simulink model "bh_4dof_LAGR_manipulator_CONTROL_PID"  (R2016b)
settings: Solver=ode15s  StartTime=0.0  StopTime=60  FixedStep=0.001  RelTol=1e-5  EnableMultiTasking=on
values from neighbouring files (symbols this model uses):
  N = 3    [bh_4dof_sim_post_process.m]
undefined symbols (not defined in the file or in its folder): b1_damp, b2_damp, b3_damp, b4_damp, g, Hz, L1x, L1y, L1z, L2x, L2y, L2z, L3x, L3y, L3z, mass1, mass2, mass3, mass4, Rturn, theta1_0, theta1_dot_0, theta2_0, theta2_dot_0, theta3_0, theta3_dot_0, theta4_0, theta4_dot_0, X, Y, Z
libraries: sm_lib x25, nesl_utility x17, simulink x9, simulink_extras x2
(part 1 of 3)
settings Model: Creator=bhorton  LastModifiedBy=bhorton
settings SolverCC: ZeroCrossAlgorithm=Adaptive
settings OptimizationCC: LifeSpan=inf
settings DebuggingCC: SFUnexpectedBacktrackingDiag=warning  SFNoUnconditionalDefaultTransitionDiag=warning  SFExecutionAtInitializationDiag=none
settings GRTTargetCC: TargetLangStandard=C89/C90 (ANSI)
settings ConfigComp: CovMetricSettings=dw  CovHtmlReporting=on  CovSaveCumulativeToWorkspaceVar=on  CovSaveSingleToWorkspaceVar=on  CovExternalEMLEnable=off
settings SimscapeCC: SimscapeLogType=all  SimscapeLogDataHistory=10000

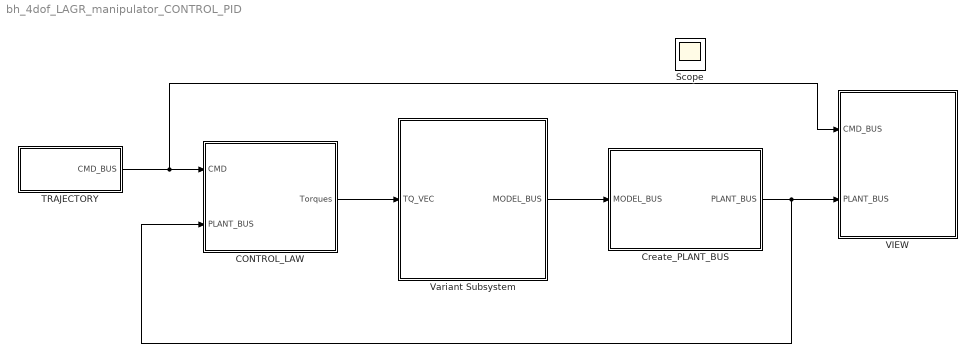
== system bh_4dof_LAGR_manipulator_CONTROL_PID ==
  CONTROL_LAW : Subsystem
  Create_PLANT_BUS : Subsystem
  TRAJECTORY : Subsystem
  VIEW : Subsystem
  Variant Subsystem : Subsystem  Variant=on  OverrideUsingVariant=Variant
  Scope : Scope
  wires:
  TRAJECTORY/1(CMD_BUS) -> VIEW/1(CMD_BUS), CONTROL_LAW/1(CMD)
  Create_PLANT_BUS/1(PLANT_BUS) -> VIEW/2(PLANT_BUS), CONTROL_LAW/2(PLANT_BUS)
  Variant Subsystem/1(MODEL_BUS) -> Create_PLANT_BUS/1(MODEL_BUS)
  CONTROL_LAW/1(Torques) -> Variant Subsystem/1(TQ_VEC)

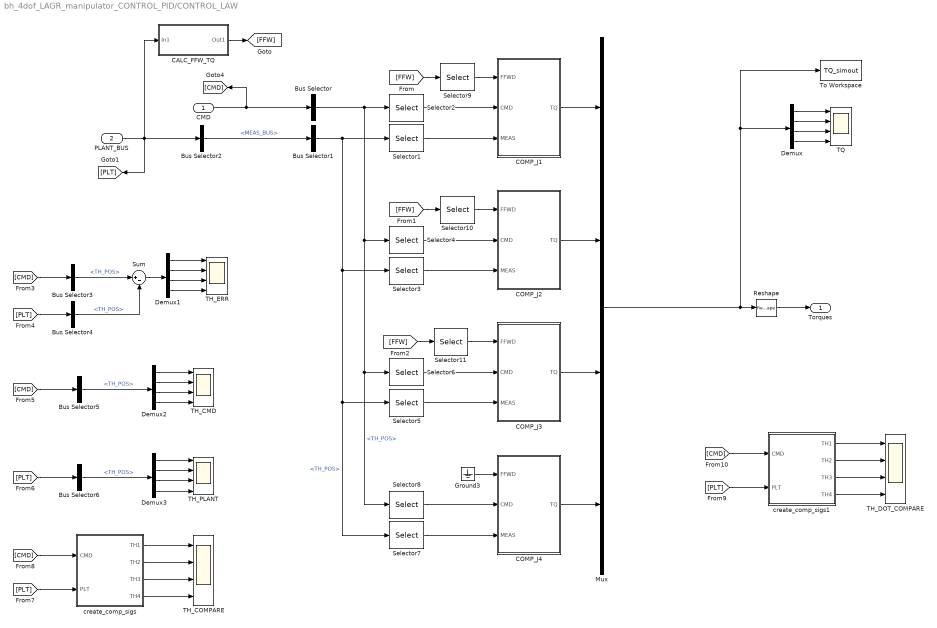
== system bh_4dof_LAGR_manipulator_CONTROL_PID/CONTROL_LAW ==
  CMD : Inport
  PLANT_BUS : Inport  Port=2
  Bus Selector{,1,3,5} (4 alike) : BusSelector  OutputSignals=TH_POS
  Bus Selector2 : BusSelector  OutputSignals=MEAS_BUS
  Bus Selector4 : BusSelector  OutputSignals=MEAS_BUS.TH_POS
  Bus Selector6 : BusSelector  OutputSignals=MEAS_BUS.TH_POS
  CALC_FFW_TQ : Subsystem
  COMP_J1 : Subsystem
  COMP_J2 : Subsystem
  COMP_J3 : Subsystem
  COMP_J4 : Subsystem
  Demux{,1..3} (4 alike) : Demux
  Ground3 : Ground
  Mux : Mux
  Reshape : Reshape  OutputDimensionality=Column vector (2-D)
  Selector1 : Selector  InputPortWidth=4  IndexOptions=Index vector (dialog)  Indices=1  OutputSizes=1
  Selector10 : Selector  InputPortWidth=3  IndexOptions=Index vector (dialog)  Indices=2  OutputSizes=1
  Selector11 : Selector  InputPortWidth=3  IndexOptions=Index vector (dialog)  Indices=3  OutputSizes=1
  Selector2 : Selector  InputPortWidth=4  IndexOptions=Index vector (dialog)  Indices=1  OutputSizes=1
  Selector3 : Selector  InputPortWidth=4  IndexOptions=Index vector (dialog)  Indices=2  OutputSizes=1
  Selector4 : Selector  InputPortWidth=4  IndexOptions=Index vector (dialog)  Indices=2  OutputSizes=1
  Selector5 : Selector  InputPortWidth=4  IndexOptions=Index vector (dialog)  Indices=3  OutputSizes=1
  Selector6 : Selector  InputPortWidth=4  IndexOptions=Index vector (dialog)  Indices=3  OutputSizes=1
  Selector7 : Selector  InputPortWidth=4  IndexOptions=Index vector (dialog)  Indices=4  OutputSizes=1
  Selector8 : Selector  InputPortWidth=4  IndexOptions=Index vector (dialog)  Indices=4  OutputSizes=1
  Selector9 : Selector  InputPortWidth=3  IndexOptions=Index vector (dialog)  Indices=1  OutputSizes=1
  Sum : Sum  Inputs=|+-
  TH_CMD : Scope  NumInputPorts=4
  TH_COMPARE : Scope  NumInputPorts=4
  TH_DOT_COMPARE : Scope  NumInputPorts=4
  TH_ERR : Scope  NumInputPorts=4
  TH_PLANT : Scope  NumInputPorts=4
  TQ : Scope  NumInputPorts=4
  To Workspace : ToWorkspace  VariableName=TQ_simout  SaveFormat=Structure With Time  SampleTime=-1
  create_comp_sigs : Subsystem
  create_comp_sigs1 : Subsystem
  Torques : Outport
  wires:
  Reshape/1 -> Torques/1
  Selector9/1 -> COMP_J1/1(FFWD)
  CMD/1 -> [CMD], Bus Selector/1
  Selector1/1 -> COMP_J1/3(MEAS)
  Selector2/1 -> COMP_J1/2(CMD)
  Bus Selector/1 -> Selector8/1, Selector6/1, Selector4/1, Selector2/1  "<TH_POS>"
  Bus Selector1/1 -> Selector5/1, Selector7/1, Selector3/1, Selector1/1  "<TH_POS>"
  Selector6/1 -> COMP_J3/2(CMD)
  Selector5/1 -> COMP_J3/3(MEAS)
  Selector3/1 -> COMP_J2/3(MEAS)
  Selector4/1 -> COMP_J2/2(CMD)
  Ground3/1 -> COMP_J4/1(FFWD)
  Selector8/1 -> COMP_J4/2(CMD)
  Selector7/1 -> COMP_J4/3(MEAS)
  COMP_J4/1(TQ) -> Mux/4
  COMP_J3/1(TQ) -> Mux/3
  COMP_J2/1(TQ) -> Mux/2
  COMP_J1/1(TQ) -> Mux/1
  Bus Selector2/1 -> Bus Selector1/1  "<MEAS_BUS>"
  Demux/1 -> TQ/1
  Demux/2 -> TQ/2
  Demux/4 -> TQ/4
  Demux/3 -> TQ/3
  CALC_FFW_TQ/1(Out1) -> [FFW]
  [FFW] -> Selector9/1
  [FFW] -> Selector10/1
  Selector10/1 -> COMP_J2/1(FFWD)
  [FFW] -> Selector11/1
  Selector11/1 -> COMP_J3/1(FFWD)
  Demux1/1 -> TH_ERR/1
  Demux1/2 -> TH_ERR/2
  Demux1/4 -> TH_ERR/4
  Demux1/3 -> TH_ERR/3
  PLANT_BUS/1 -> [PLT], CALC_FFW_TQ/1(In1), Bus Selector2/1
  [CMD] -> Bus Selector3/1
  [PLT] -> Bus Selector4/1
  Bus Selector3/1 -> Sum/1  "<TH_POS>"
  Bus Selector4/1 -> Sum/2  "<TH_POS>"
  Sum/1 -> Demux1/1
  Demux2/1 -> TH_CMD/1
  Demux2/2 -> TH_CMD/2
  Demux2/4 -> TH_CMD/4
  Demux2/3 -> TH_CMD/3
  [CMD] -> Bus Selector5/1
  Bus Selector5/1 -> Demux2/1  "<TH_POS>"
  Demux3/1 -> TH_PLANT/1
  Demux3/2 -> TH_PLANT/2
  Demux3/4 -> TH_PLANT/4
  Demux3/3 -> TH_PLANT/3
  [PLT] -> Bus Selector6/1
  Bus Selector6/1 -> Demux3/1  "<TH_POS>"
  [PLT] -> create_comp_sigs/2(PLT)
  [CMD] -> create_comp_sigs/1(CMD)
  create_comp_sigs/1(TH1) -> TH_COMPARE/1
  create_comp_sigs/2(TH2) -> TH_COMPARE/2
  create_comp_sigs/3(TH3) -> TH_COMPARE/3
  create_comp_sigs/4(TH4) -> TH_COMPARE/4
  [PLT] -> create_comp_sigs1/2(PLT)
  [CMD] -> create_comp_sigs1/1(CMD)
  create_comp_sigs1/1(TH1) -> TH_DOT_COMPARE/1
  create_comp_sigs1/2(TH2) -> TH_DOT_COMPARE/2
  create_comp_sigs1/3(TH3) -> TH_DOT_COMPARE/3
  create_comp_sigs1/4(TH4) -> TH_DOT_COMPARE/4
  Mux/1 -> To Workspace/1, Demux/1, Reshape/1

== system bh_4dof_LAGR_manipulator_CONTROL_PID/Create_PLANT_BUS ==
  MODEL_BUS : Inport
  CALC_BUS : Subsystem
  MEAS : Subsystem
  Subsystem : Subsystem
  Subsystem1 : Subsystem
  PLANT_BUS : Outport
  wires:
  MODEL_BUS/1 -> MEAS/1(MODEL_BUS), CALC_BUS/1(MODEL_BUS), Subsystem/1(MODEL)
  Subsystem/1(PLANT_B) -> PLANT_BUS/1
  CALC_BUS/1(CALC_POS) -> Subsystem1/1(POS), Subsystem/3(CALC_POS)
  MEAS/1(MEAS) -> Subsystem/2(MEAS)
  Subsystem1/1(GTQ) -> Subsystem/4(CALC_GRAV_TQ)

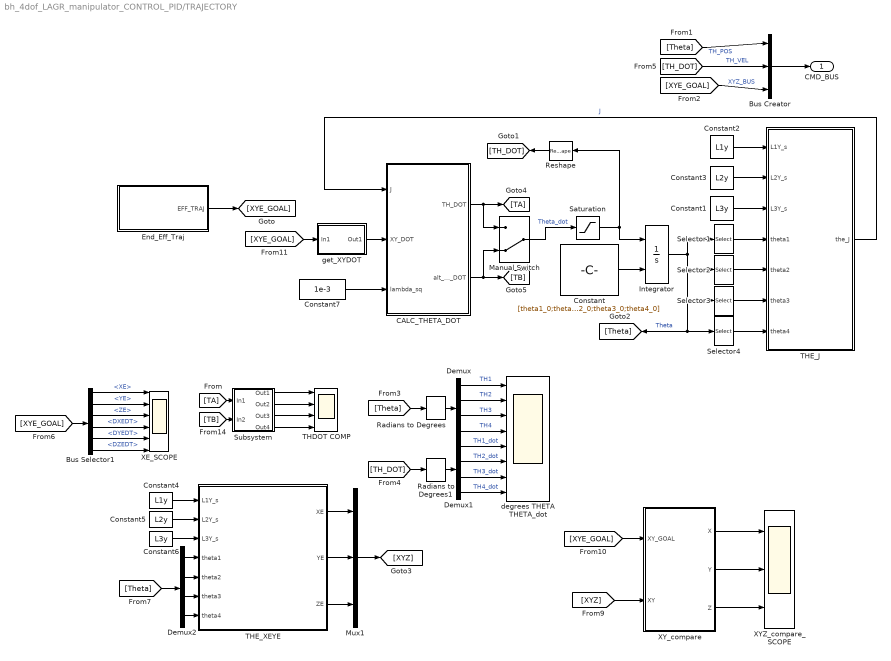
== system bh_4dof_LAGR_manipulator_CONTROL_PID/TRAJECTORY ==
  Bus Creator : BusCreator  Inputs=3
  Bus Selector1 : BusSelector  OutputSignals=XE,YE,ZE,DXEDT,DYEDT,DZEDT
  CALC_THETA_DOT : MATLAB Function  TreatAsAtomicUnit=on
  Constant : Constant  Value=[theta1_0;theta2_0;theta3_0;theta4_0]  VectorParams1D=off
  Constant1 : Constant  Value=L3y
  Constant2 : Constant  Value=L1y
  Constant3 : Constant  Value=L2y
  Constant4 : Constant  Value=L1y
  Constant5 : Constant  Value=L2y
  Constant6 : Constant  Value=L3y
  Constant7 : Constant  Value=1e-3
  Demux : Demux
  Demux1 : Demux
  Demux2 : Demux
  End_Eff_Traj : Subsystem
  Integrator : Integrator  InitialConditionSource=external
  Manual Switch : ManualSwitch  CurrentSetting=0
  Mux1 : Mux  Inputs=3
  Radians to Degrees : simulink_extras/Transformations/Radians to Degrees
  Radians to Degrees1 : simulink_extras/Transformations/Radians to Degrees
  Reshape : Reshape  OutputDimensionality=Column vector (2-D)
  Saturation : Saturate  UpperLimit=6  LowerLimit=-6
  Selector1 : Selector  InputPortWidth=4  IndexOptions=Index vector (dialog)  Indices=1  OutputSizes=1
  Selector2 : Selector  InputPortWidth=4  IndexOptions=Index vector (dialog)  Indices=2  OutputSizes=1
  Selector3 : Selector  InputPortWidth=4  IndexOptions=Index vector (dialog)  Indices=3  OutputSizes=1
  Selector4 : Selector  InputPortWidth=4  IndexOptions=Index vector (dialog)  Indices=4  OutputSizes=1
  Subsystem : Subsystem
  THDOT COMP : Scope  NumInputPorts=4
  THE_J : MATLAB Function  TreatAsAtomicUnit=on
  THE_XEYE : MATLAB Function  TreatAsAtomicUnit=on
  XE_SCOPE : Scope  NumInputPorts=6
  XYZ_compare_SCOPE : Scope  NumInputPorts=3
  XY_compare : Subsystem
  degrees THETA THETA_dot : Scope  NumInputPorts=8
  get_XYDOT : Subsystem
  CMD_BUS : Outport
  wires:
  Bus Selector1/1 -> XE_SCOPE/1  "<XE>"
  Bus Selector1/2 -> XE_SCOPE/2  "<YE>"
  Bus Selector1/3 -> XE_SCOPE/3  "<ZE>"
  Bus Selector1/4 -> XE_SCOPE/4  "<DXEDT>"
  Bus Selector1/5 -> XE_SCOPE/5  "<DYEDT>"
  Bus Selector1/6 -> XE_SCOPE/6  "<DZEDT>"
  [XYE_GOAL] -> Bus Selector1/1
  Constant/1 -> Integrator/2
  THE_J/1(the_J) -> CALC_THETA_DOT/1(J)  "J"
  get_XYDOT/1(Out1) -> CALC_THETA_DOT/2(XY_DOT)
  Manual Switch/1 -> Saturation/1  "Theta_dot"
  Integrator/1 -> Selector4/1, [Theta], Selector3/1, Selector2/1, Selector1/1  "Theta"
  [XYE_GOAL] -> get_XYDOT/1(In1)
  Saturation/1 -> Integrator/1, Reshape/1
  Selector4/1 -> THE_J/7(theta4)
  Selector3/1 -> THE_J/6(theta3)
  Selector2/1 -> THE_J/5(theta2)
  Selector1/1 -> THE_J/4(theta1)
  Constant2/1 -> THE_J/1(L1Y_s)
  Constant3/1 -> THE_J/2(L2Y_s)
  Constant1/1 -> THE_J/3(L3Y_s)
  CALC_THETA_DOT/1(TH_DOT) -> [TA], Manual Switch/1
  CALC_THETA_DOT/2(alt_TH_DOT) -> [TB], Manual Switch/2
  Constant7/1 -> CALC_THETA_DOT/3(lambda_sq)
  [TB] -> Subsystem/2(In2)
  [TA] -> Subsystem/1(In1)
  Subsystem/1(Out1) -> THDOT COMP/1
  Subsystem/2(Out2) -> THDOT COMP/2
  Subsystem/3(Out3) -> THDOT COMP/3
  Subsystem/4(Out4) -> THDOT COMP/4
  End_Eff_Traj/1(EFF_TRAJ) -> [XYE_GOAL]
  [TH_DOT] -> Bus Creator/2  "TH_VEL"
  [Theta] -> Bus Creator/1  "TH_POS"
  Bus Creator/1 -> CMD_BUS/1
  Reshape/1 -> [TH_DOT]
  [XYE_GOAL] -> Bus Creator/3  "XYZ_BUS"
  Demux/4 -> degrees THETA THETA_dot/4  "TH4"
  Demux/3 -> degrees THETA THETA_dot/3  "TH3"
  Demux/2 -> degrees THETA THETA_dot/2  "TH2"
  Demux/1 -> degrees THETA THETA_dot/1  "TH1"
  Demux1/1 -> degrees THETA THETA_dot/5  "TH1_dot"
  Demux1/2 -> degrees THETA THETA_dot/6  "TH2_dot"
  Demux1/3 -> degrees THETA THETA_dot/7  "TH3_dot"
  Demux1/4 -> degrees THETA THETA_dot/8  "TH4_dot"
  [Theta] -> Radians to Degrees/1
  Radians to Degrees/1 -> Demux/1
  [TH_DOT] -> Radians to Degrees1/1
  Radians to Degrees1/1 -> Demux1/1
  Constant4/1 -> THE_XEYE/1(L1Y_s)
  Constant6/1 -> THE_XEYE/3(L3Y_s)
  Constant5/1 -> THE_XEYE/2(L2Y_s)
  Demux2/1 -> THE_XEYE/4(theta1)
  Demux2/2 -> THE_XEYE/5(theta2)
  Demux2/3 -> THE_XEYE/6(theta3)
  Demux2/4 -> THE_XEYE/7(theta4)
  [Theta] -> Demux2/1
  THE_XEYE/1(XE) -> Mux1/1
  THE_XEYE/3(ZE) -> Mux1/3
  THE_XEYE/2(YE) -> Mux1/2
  Mux1/1 -> [XYZ]
  [XYZ] -> XY_compare/2(XY)
  XY_compare/2(Y) -> XYZ_compare_SCOPE/2
  XY_compare/1(X) -> XYZ_compare_SCOPE/1
  [XYE_GOAL] -> XY_compare/1(XY_GOAL)
  XY_compare/3(Z) -> XYZ_compare_SCOPE/3

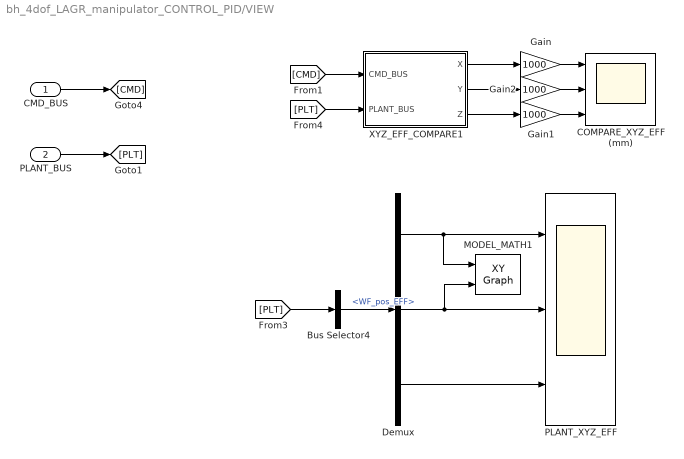
== system bh_4dof_LAGR_manipulator_CONTROL_PID/VIEW ==
  CMD_BUS : Inport
  PLANT_BUS : Inport  Port=2
  Bus Selector4 : BusSelector  OutputSignals=CALC_POS_BUS.WF_pos_EFF
  COMPARE_XYZ_EFF (mm) : Scope  NumInputPorts=3
  Demux : Demux  Outputs=3
  Gain : Gain  Gain=1000
  Gain1 : Gain  Gain=1000
  Gain2 : Gain  Gain=1000
  MODEL_MATH1 : simulink/Sinks/XY Graph  xmin=0  xmax=1.6  ymin=0  ymax=1.6  st=-1
  PLANT_XYZ_EFF : Scope  NumInputPorts=3
  XYZ_EFF_COMPARE1 : Subsystem
  wires:
  CMD_BUS/1 -> [CMD]
  PLANT_BUS/1 -> [PLT]
  Bus Selector4/1 -> Demux/1  "<WF_pos_EFF>"
  Demux/1 -> MODEL_MATH1/1, PLANT_XYZ_EFF/1
  Demux/2 -> MODEL_MATH1/2, PLANT_XYZ_EFF/2
  [PLT] -> Bus Selector4/1
  Demux/3 -> PLANT_XYZ_EFF/3
  [CMD] -> XYZ_EFF_COMPARE1/1(CMD_BUS)
  [PLT] -> XYZ_EFF_COMPARE1/2(PLANT_BUS)
  XYZ_EFF_COMPARE1/1(X) -> Gain/1
  XYZ_EFF_COMPARE1/2(Y) -> Gain2/1
  XYZ_EFF_COMPARE1/3(Z) -> Gain1/1
  Gain/1 -> COMPARE_XYZ_EFF (mm)/1
  Gain1/1 -> COMPARE_XYZ_EFF (mm)/3
  Gain2/1 -> COMPARE_XYZ_EFF (mm)/2

== system bh_4dof_LAGR_manipulator_CONTROL_PID/Variant Subsystem ==
  note: 1) Add Subsystem or Model blocks as valid variant choices.
      | 2) You cannot connect blocks at this level. At simulation, connectivity is automatically
      | determined, based on the active variant and port name matching.
  TQ_VEC : Inport
  SIMSCAPE : Subsystem  VariantControl=Variant
  SIMULINK_MODEL : Subsystem  VariantControl=Variant1
  MODEL_BUS : Outport

== system bh_4dof_LAGR_manipulator_CONTROL_PID/CONTROL_LAW/CALC_FFW_TQ ==
  In1 : Inport
  Bus Selector1 : BusSelector  OutputSignals=TQ_GRAV_at_JOINT_1,TQ_GRAV_at_JOINT_2,TQ_GRAV_at_JOINT_3
  Bus Selector2 : BusSelector  OutputSignals=CALC_GRAV_TQ_BUS
  Constant : Constant  Value=0
  Gain1 : Gain  Gain=-1
  Gain2 : Gain  Gain=-1
  Gain3 : Gain  Gain=-1
  Manual Switch : ManualSwitch  CurrentSetting=0
  Mux : Mux  Inputs=3
  Mux1 : Mux  Inputs=3
  Out1 : Outport
  wires:
  In1/1 -> Bus Selector2/1
  Bus Selector2/1 -> Bus Selector1/1  "<CALC_GRAV_TQ_BUS>"
  Bus Selector1/1 -> Gain1/1  "<TQ_GRAV_at_JOINT_1>"
  Bus Selector1/2 -> Gain2/1  "<TQ_GRAV_at_JOINT_2>"
  Bus Selector1/3 -> Gain3/1  "<TQ_GRAV_at_JOINT_3>"
  Gain1/1 -> Mux/1
  Gain2/1 -> Mux/2
  Gain3/1 -> Mux/3
  Constant/1 -> Mux1/3, Mux1/2, Mux1/1
  Mux/1 -> Manual Switch/1
  Mux1/1 -> Manual Switch/2
  Manual Switch/1 -> Out1/1

== system bh_4dof_LAGR_manipulator_CONTROL_PID/CONTROL_LAW/COMP_J1 ==
  FFWD : Inport
  CMD : Inport  Port=2
  MEAS : Inport  Port=3
  PID Controller : simulink/Continuous/PID Controller  Controller=PID  TimeDomain=Continuous-time  SampleTime=-1  IntegratorMethod=Forward Euler  FilterMethod=Forward Euler  Form=Parallel  UseFilter=on  ControllerParametersSource=internal  P=96.7963776447224  I=147.314632554553  D=14.1316637412563  N=29813.0572073536  InitialConditionSource=internal  InitialConditionForIntegrator=0  InitialConditionForFilter=0  ExternalReset=none  LimitOutput=off  UpperSaturationLimit=inf  LowerSaturationLimit=-inf  LinearizeAsGain=on  AntiWindupMode=none  Kb=1  TrackingMode=off  Kt=1  PParamMin=[]  PParamMax=[]  IParamMin=[]  IParamMax=[]  DParamMin=[]  DParamMax=[]  NParamMin=[]  NParamMax=[]  KbParamMin=[]  KbParamMax=[]  KtParamMin=[]  KtParamMax=[]  POutMin=[]  POutMax=[]  IOutMin=[]  IOutMax=[]  DOutMin=[]  DOutMax=[]  NOutMin=[]  NOutMax=[]  KbOutMin=[]  KbOutMax=[]  KtOutMin=[]  KtOutMax=[]  IntegratorOutMin=[]  IntegratorOutMax=[]  FilterOutMin=[]  FilterOutMax=[]  SumOutMin=[]  SumOutMax=[]  SumI1OutMin=[]  SumI1OutMax=[]  SumI2OutMin=[]  SumI2OutMax=[]  SumI3OutMin=[]  SumI3OutMax=[]  SumDOutMin=[]  SumDOutMax=[]  SaturationOutMin=[]  SaturationOutMax=[]  IntegratorContinuousStateAttributes=''  IntegratorStateMustResolveToSignalObject=off  IntegratorRTWStateStorageClass=Auto  FilterContinuousStateAttributes=''  FilterStateMustResolveToSignalObject=off  FilterRTWStateStorageClass=Auto  DifferentiatorICPrevScaledInput=0  DifferentiatorOutMin=[]  DifferentiatorOutMax=[]
  PID Controller1 : simulink/Continuous/PID Controller  Commented=on  Controller=PID  TimeDomain=Continuous-time  SampleTime=-1  IntegratorMethod=Forward Euler  FilterMethod=Forward Euler  Form=Parallel  UseFilter=on  ControllerParametersSource=internal  P=1  I=1  D=0  N=100  InitialConditionSource=internal  InitialConditionForIntegrator=0  InitialConditionForFilter=0  ExternalReset=none  LimitOutput=off  UpperSaturationLimit=inf  LowerSaturationLimit=-inf  LinearizeAsGain=on  AntiWindupMode=none  Kb=1  TrackingMode=off  Kt=1  PParamMin=[]  PParamMax=[]  IParamMin=[]  IParamMax=[]  DParamMin=[]  DParamMax=[]  NParamMin=[]  NParamMax=[]  KbParamMin=[]  KbParamMax=[]  KtParamMin=[]  KtParamMax=[]  POutMin=[]  POutMax=[]  IOutMin=[]  IOutMax=[]  DOutMin=[]  DOutMax=[]  NOutMin=[]  NOutMax=[]  KbOutMin=[]  KbOutMax=[]  KtOutMin=[]  KtOutMax=[]  IntegratorOutMin=[]  IntegratorOutMax=[]  FilterOutMin=[]  FilterOutMax=[]  SumOutMin=[]  SumOutMax=[]  SumI1OutMin=[]  SumI1OutMax=[]  SumI2OutMin=[]  SumI2OutMax=[]  SumI3OutMin=[]  SumI3OutMax=[]  SumDOutMin=[]  SumDOutMax=[]  SaturationOutMin=[]  SaturationOutMax=[]  IntegratorContinuousStateAttributes=''  IntegratorStateMustResolveToSignalObject=off  IntegratorRTWStateStorageClass=Auto  FilterContinuousStateAttributes=''  FilterStateMustResolveToSignalObject=off  FilterRTWStateStorageClass=Auto  DifferentiatorICPrevScaledInput=0  DifferentiatorOutMin=[]  DifferentiatorOutMax=[]
  Sum : Sum  Inputs=|+-
  Sum1 : Sum  Inputs=++|
  TQ : Outport
  wires:
  CMD/1 -> Sum/1
  MEAS/1 -> Sum/2
  Sum1/1 -> TQ/1
  FFWD/1 -> Sum1/1
  Sum/1 -> PID Controller/1
  PID Controller/1 -> Sum1/2

== system bh_4dof_LAGR_manipulator_CONTROL_PID/CONTROL_LAW/COMP_J2 ==
  FFWD : Inport
  CMD : Inport  Port=2
  MEAS : Inport  Port=3
  PID Controller : simulink/Continuous/PID Controller  Controller=PID  TimeDomain=Continuous-time  SampleTime=-1  IntegratorMethod=Forward Euler  FilterMethod=Forward Euler  Form=Parallel  UseFilter=on  ControllerParametersSource=internal  P=1118.27053440134  I=29767.9762659611  D=6.3323395620565  N=172364.631443819  InitialConditionSource=internal  InitialConditionForIntegrator=0  InitialConditionForFilter=0  ExternalReset=none  LimitOutput=off  UpperSaturationLimit=inf  LowerSaturationLimit=-inf  LinearizeAsGain=on  AntiWindupMode=none  Kb=1  TrackingMode=off  Kt=1  PParamMin=[]  PParamMax=[]  IParamMin=[]  IParamMax=[]  DParamMin=[]  DParamMax=[]  NParamMin=[]  NParamMax=[]  KbParamMin=[]  KbParamMax=[]  KtParamMin=[]  KtParamMax=[]  POutMin=[]  POutMax=[]  IOutMin=[]  IOutMax=[]  DOutMin=[]  DOutMax=[]  NOutMin=[]  NOutMax=[]  KbOutMin=[]  KbOutMax=[]  KtOutMin=[]  KtOutMax=[]  IntegratorOutMin=[]  IntegratorOutMax=[]  FilterOutMin=[]  FilterOutMax=[]  SumOutMin=[]  SumOutMax=[]  SumI1OutMin=[]  SumI1OutMax=[]  SumI2OutMin=[]  SumI2OutMax=[]  SumI3OutMin=[]  SumI3OutMax=[]  SumDOutMin=[]  SumDOutMax=[]  SaturationOutMin=[]  SaturationOutMax=[]  IntegratorContinuousStateAttributes=''  IntegratorStateMustResolveToSignalObject=off  IntegratorRTWStateStorageClass=Auto  FilterContinuousStateAttributes=''  FilterStateMustResolveToSignalObject=off  FilterRTWStateStorageClass=Auto  DifferentiatorICPrevScaledInput=0  DifferentiatorOutMin=[]  DifferentiatorOutMax=[]
  PID Controller1 : simulink/Continuous/PID Controller  Commented=on  Controller=PID  TimeDomain=Continuous-time  SampleTime=-1  IntegratorMethod=Forward Euler  FilterMethod=Forward Euler  Form=Parallel  UseFilter=on  ControllerParametersSource=internal  P=1  I=1  D=0  N=100  InitialConditionSource=internal  InitialConditionForIntegrator=0  InitialConditionForFilter=0  ExternalReset=none  LimitOutput=off  UpperSaturationLimit=inf  LowerSaturationLimit=-inf  LinearizeAsGain=on  AntiWindupMode=none  Kb=1  TrackingMode=off  Kt=1  PParamMin=[]  PParamMax=[]  IParamMin=[]  IParamMax=[]  DParamMin=[]  DParamMax=[]  NParamMin=[]  NParamMax=[]  KbParamMin=[]  KbParamMax=[]  KtParamMin=[]  KtParamMax=[]  POutMin=[]  POutMax=[]  IOutMin=[]  IOutMax=[]  DOutMin=[]  DOutMax=[]  NOutMin=[]  NOutMax=[]  KbOutMin=[]  KbOutMax=[]  KtOutMin=[]  KtOutMax=[]  IntegratorOutMin=[]  IntegratorOutMax=[]  FilterOutMin=[]  FilterOutMax=[]  SumOutMin=[]  SumOutMax=[]  SumI1OutMin=[]  SumI1OutMax=[]  SumI2OutMin=[]  SumI2OutMax=[]  SumI3OutMin=[]  SumI3OutMax=[]  SumDOutMin=[]  SumDOutMax=[]  SaturationOutMin=[]  SaturationOutMax=[]  IntegratorContinuousStateAttributes=''  IntegratorStateMustResolveToSignalObject=off  IntegratorRTWStateStorageClass=Auto  FilterContinuousStateAttributes=''  FilterStateMustResolveToSignalObject=off  FilterRTWStateStorageClass=Auto  DifferentiatorICPrevScaledInput=0  DifferentiatorOutMin=[]  DifferentiatorOutMax=[]
  Sum : Sum  Inputs=|+-
  Sum1 : Sum  Inputs=++|
  TQ : Outport
  wires:
  CMD/1 -> Sum/1
  MEAS/1 -> Sum/2
  Sum1/1 -> TQ/1
  FFWD/1 -> Sum1/1
  Sum/1 -> PID Controller/1
  PID Controller/1 -> Sum1/2

== system bh_4dof_LAGR_manipulator_CONTROL_PID/CONTROL_LAW/COMP_J3 ==
  FFWD : Inport
  CMD : Inport  Port=2
  MEAS : Inport  Port=3
  PID Controller : simulink/Continuous/PID Controller  Controller=PID  TimeDomain=Continuous-time  SampleTime=-1  IntegratorMethod=Forward Euler  FilterMethod=Forward Euler  Form=Parallel  UseFilter=on  ControllerParametersSource=internal  P=11621.8887294897  I=2067489.49327814  D=14.515469457271  N=3484867.97953316  InitialConditionSource=internal  InitialConditionForIntegrator=0  InitialConditionForFilter=0  ExternalReset=none  LimitOutput=off  UpperSaturationLimit=inf  LowerSaturationLimit=-inf  LinearizeAsGain=on  AntiWindupMode=none  Kb=1  TrackingMode=off  Kt=1  PParamMin=[]  PParamMax=[]  IParamMin=[]  IParamMax=[]  DParamMin=[]  DParamMax=[]  NParamMin=[]  NParamMax=[]  KbParamMin=[]  KbParamMax=[]  KtParamMin=[]  KtParamMax=[]  POutMin=[]  POutMax=[]  IOutMin=[]  IOutMax=[]  DOutMin=[]  DOutMax=[]  NOutMin=[]  NOutMax=[]  KbOutMin=[]  KbOutMax=[]  KtOutMin=[]  KtOutMax=[]  IntegratorOutMin=[]  IntegratorOutMax=[]  FilterOutMin=[]  FilterOutMax=[]  SumOutMin=[]  SumOutMax=[]  SumI1OutMin=[]  SumI1OutMax=[]  SumI2OutMin=[]  SumI2OutMax=[]  SumI3OutMin=[]  SumI3OutMax=[]  SumDOutMin=[]  SumDOutMax=[]  SaturationOutMin=[]  SaturationOutMax=[]  IntegratorContinuousStateAttributes=''  IntegratorStateMustResolveToSignalObject=off  IntegratorRTWStateStorageClass=Auto  FilterContinuousStateAttributes=''  FilterStateMustResolveToSignalObject=off  FilterRTWStateStorageClass=Auto  DifferentiatorICPrevScaledInput=0  DifferentiatorOutMin=[]  DifferentiatorOutMax=[]
  PID Controller1 : simulink/Continuous/PID Controller  Commented=on  Controller=PID  TimeDomain=Continuous-time  SampleTime=-1  IntegratorMethod=Forward Euler  FilterMethod=Forward Euler  Form=Parallel  UseFilter=on  ControllerParametersSource=internal  P=1  I=1  D=0  N=100  InitialConditionSource=internal  InitialConditionForIntegrator=0  InitialConditionForFilter=0  ExternalReset=none  LimitOutput=off  UpperSaturationLimit=inf  LowerSaturationLimit=-inf  LinearizeAsGain=on  AntiWindupMode=none  Kb=1  TrackingMode=off  Kt=1  PParamMin=[]  PParamMax=[]  IParamMin=[]  IParamMax=[]  DParamMin=[]  DParamMax=[]  NParamMin=[]  NParamMax=[]  KbParamMin=[]  KbParamMax=[]  KtParamMin=[]  KtParamMax=[]  POutMin=[]  POutMax=[]  IOutMin=[]  IOutMax=[]  DOutMin=[]  DOutMax=[]  NOutMin=[]  NOutMax=[]  KbOutMin=[]  KbOutMax=[]  KtOutMin=[]  KtOutMax=[]  IntegratorOutMin=[]  IntegratorOutMax=[]  FilterOutMin=[]  FilterOutMax=[]  SumOutMin=[]  SumOutMax=[]  SumI1OutMin=[]  SumI1OutMax=[]  SumI2OutMin=[]  SumI2OutMax=[]  SumI3OutMin=[]  SumI3OutMax=[]  SumDOutMin=[]  SumDOutMax=[]  SaturationOutMin=[]  SaturationOutMax=[]  IntegratorContinuousStateAttributes=''  IntegratorStateMustResolveToSignalObject=off  IntegratorRTWStateStorageClass=Auto  FilterContinuousStateAttributes=''  FilterStateMustResolveToSignalObject=off  FilterRTWStateStorageClass=Auto  DifferentiatorICPrevScaledInput=0  DifferentiatorOutMin=[]  DifferentiatorOutMax=[]
  Sum : Sum  Inputs=|+-
  Sum1 : Sum  Inputs=++|
  TQ : Outport
  wires:
  CMD/1 -> Sum/1
  MEAS/1 -> Sum/2
  Sum1/1 -> TQ/1
  FFWD/1 -> Sum1/1
  Sum/1 -> PID Controller/1
  PID Controller/1 -> Sum1/2

== system bh_4dof_LAGR_manipulator_CONTROL_PID/CONTROL_LAW/COMP_J4 ==
  FFWD : Inport
  CMD : Inport  Port=2
  MEAS : Inport  Port=3
  PID Controller : simulink/Continuous/PID Controller  Controller=PID  TimeDomain=Continuous-time  SampleTime=-1  IntegratorMethod=Forward Euler  FilterMethod=Forward Euler  Form=Parallel  UseFilter=on  ControllerParametersSource=internal  P=1277.12722924899  I=3088.28849566436  D=117.346850130911  N=47370.0050500609  InitialConditionSource=internal  InitialConditionForIntegrator=0  InitialConditionForFilter=0  ExternalReset=none  LimitOutput=off  UpperSaturationLimit=inf  LowerSaturationLimit=-inf  LinearizeAsGain=on  AntiWindupMode=none  Kb=1  TrackingMode=off  Kt=1  PParamMin=[]  PParamMax=[]  IParamMin=[]  IParamMax=[]  DParamMin=[]  DParamMax=[]  NParamMin=[]  NParamMax=[]  KbParamMin=[]  KbParamMax=[]  KtParamMin=[]  KtParamMax=[]  POutMin=[]  POutMax=[]  IOutMin=[]  IOutMax=[]  DOutMin=[]  DOutMax=[]  NOutMin=[]  NOutMax=[]  KbOutMin=[]  KbOutMax=[]  KtOutMin=[]  KtOutMax=[]  IntegratorOutMin=[]  IntegratorOutMax=[]  FilterOutMin=[]  FilterOutMax=[]  SumOutMin=[]  SumOutMax=[]  SumI1OutMin=[]  SumI1OutMax=[]  SumI2OutMin=[]  SumI2OutMax=[]  SumI3OutMin=[]  SumI3OutMax=[]  SumDOutMin=[]  SumDOutMax=[]  SaturationOutMin=[]  SaturationOutMax=[]  IntegratorContinuousStateAttributes=''  IntegratorStateMustResolveToSignalObject=off  IntegratorRTWStateStorageClass=Auto  FilterContinuousStateAttributes=''  FilterStateMustResolveToSignalObject=off  FilterRTWStateStorageClass=Auto  DifferentiatorICPrevScaledInput=0  DifferentiatorOutMin=[]  DifferentiatorOutMax=[]
  PID Controller1 : simulink/Continuous/PID Controller  Commented=on  Controller=PID  TimeDomain=Continuous-time  SampleTime=-1  IntegratorMethod=Forward Euler  FilterMethod=Forward Euler  Form=Parallel  UseFilter=on  ControllerParametersSource=internal  P=1  I=1  D=0  N=100  InitialConditionSource=internal  InitialConditionForIntegrator=0  InitialConditionForFilter=0  ExternalReset=none  LimitOutput=off  UpperSaturationLimit=inf  LowerSaturationLimit=-inf  LinearizeAsGain=on  AntiWindupMode=none  Kb=1  TrackingMode=off  Kt=1  PParamMin=[]  PParamMax=[]  IParamMin=[]  IParamMax=[]  DParamMin=[]  DParamMax=[]  NParamMin=[]  NParamMax=[]  KbParamMin=[]  KbParamMax=[]  KtParamMin=[]  KtParamMax=[]  POutMin=[]  POutMax=[]  IOutMin=[]  IOutMax=[]  DOutMin=[]  DOutMax=[]  NOutMin=[]  NOutMax=[]  KbOutMin=[]  KbOutMax=[]  KtOutMin=[]  KtOutMax=[]  IntegratorOutMin=[]  IntegratorOutMax=[]  FilterOutMin=[]  FilterOutMax=[]  SumOutMin=[]  SumOutMax=[]  SumI1OutMin=[]  SumI1OutMax=[]  SumI2OutMin=[]  SumI2OutMax=[]  SumI3OutMin=[]  SumI3OutMax=[]  SumDOutMin=[]  SumDOutMax=[]  SaturationOutMin=[]  SaturationOutMax=[]  IntegratorContinuousStateAttributes=''  IntegratorStateMustResolveToSignalObject=off  IntegratorRTWStateStorageClass=Auto  FilterContinuousStateAttributes=''  FilterStateMustResolveToSignalObject=off  FilterRTWStateStorageClass=Auto  DifferentiatorICPrevScaledInput=0  DifferentiatorOutMin=[]  DifferentiatorOutMax=[]
  Sum : Sum  Inputs=|+-
  Sum1 : Sum  Inputs=++|
  TQ : Outport
  wires:
  CMD/1 -> Sum/1
  MEAS/1 -> Sum/2
  Sum1/1 -> TQ/1
  FFWD/1 -> Sum1/1
  Sum/1 -> PID Controller/1
  PID Controller/1 -> Sum1/2

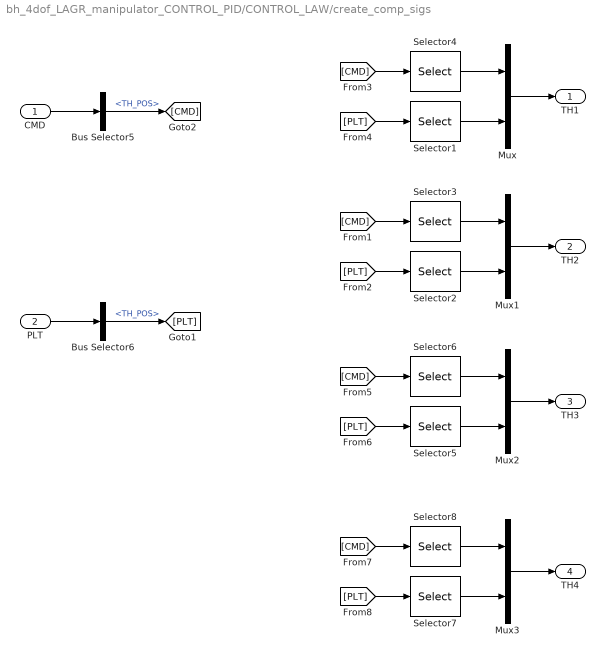
== system bh_4dof_LAGR_manipulator_CONTROL_PID/CONTROL_LAW/create_comp_sigs ==
  CMD : Inport
  PLT : Inport  Port=2
  Bus Selector5 : BusSelector  OutputSignals=TH_POS
  Bus Selector6 : BusSelector  OutputSignals=MEAS_BUS.TH_POS
  Mux{,1..3} (4 alike) : Mux  Inputs=2
  Selector1 : Selector  InputPortWidth=4  IndexOptions=Index vector (dialog)  Indices=1  OutputSizes=1
  Selector2 : Selector  InputPortWidth=4  IndexOptions=Index vector (dialog)  Indices=2  OutputSizes=1
  Selector3 : Selector  InputPortWidth=4  IndexOptions=Index vector (dialog)  Indices=2  OutputSizes=1
  Selector4 : Selector  InputPortWidth=4  IndexOptions=Index vector (dialog)  Indices=1  OutputSizes=1
  Selector5 : Selector  InputPortWidth=4  IndexOptions=Index vector (dialog)  Indices=3  OutputSizes=1
  Selector6 : Selector  InputPortWidth=4  IndexOptions=Index vector (dialog)  Indices=3  OutputSizes=1
  Selector7 : Selector  InputPortWidth=4  IndexOptions=Index vector (dialog)  Indices=4  OutputSizes=1
  Selector8 : Selector  InputPortWidth=4  IndexOptions=Index vector (dialog)  Indices=4  OutputSizes=1
  TH1 : Outport
  TH2 : Outport  Port=2
  TH3 : Outport  Port=3
  TH4 : Outport  Port=4
  wires:
  PLT/1 -> Bus Selector6/1
  Bus Selector6/1 -> [PLT]  "<TH_POS>"
  CMD/1 -> Bus Selector5/1
  Bus Selector5/1 -> [CMD]  "<TH_POS>"
  [CMD] -> Selector4/1
  Selector1/1 -> Mux/2
  Selector4/1 -> Mux/1
  [PLT] -> Selector1/1
  Mux/1 -> TH1/1
  [CMD] -> Selector3/1
  Selector2/1 -> Mux1/2
  Selector3/1 -> Mux1/1
  [PLT] -> Selector2/1
  Mux1/1 -> TH2/1
  [CMD] -> Selector6/1
  Selector5/1 -> Mux2/2
  Selector6/1 -> Mux2/1
  [PLT] -> Selector5/1
  Mux2/1 -> TH3/1
  [CMD] -> Selector8/1
  Selector7/1 -> Mux3/2
  Selector8/1 -> Mux3/1
  [PLT] -> Selector7/1
  Mux3/1 -> TH4/1

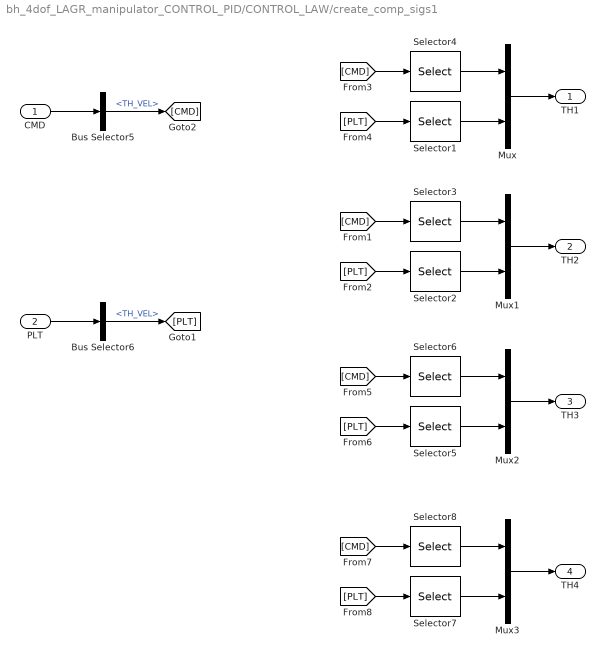
== system bh_4dof_LAGR_manipulator_CONTROL_PID/CONTROL_LAW/create_comp_sigs1 ==
  CMD : Inport
  PLT : Inport  Port=2
  Bus Selector5 : BusSelector  OutputSignals=TH_VEL
  Bus Selector6 : BusSelector  OutputSignals=MEAS_BUS.TH_VEL
  Mux{,1..3} (4 alike) : Mux  Inputs=2
  Selector1 : Selector  InputPortWidth=4  IndexOptions=Index vector (dialog)  Indices=1  OutputSizes=1
  Selector2 : Selector  InputPortWidth=4  IndexOptions=Index vector (dialog)  Indices=2  OutputSizes=1
  Selector3 : Selector  InputPortWidth=4  IndexOptions=Index vector (dialog)  Indices=2  OutputSizes=1
  Selector4 : Selector  InputPortWidth=4  IndexOptions=Index vector (dialog)  Indices=1  OutputSizes=1
  Selector5 : Selector  InputPortWidth=4  IndexOptions=Index vector (dialog)  Indices=3  OutputSizes=1
  Selector6 : Selector  InputPortWidth=4  IndexOptions=Index vector (dialog)  Indices=3  OutputSizes=1
  Selector7 : Selector  InputPortWidth=4  IndexOptions=Index vector (dialog)  Indices=4  OutputSizes=1
  Selector8 : Selector  InputPortWidth=4  IndexOptions=Index vector (dialog)  Indices=4  OutputSizes=1
  TH1 : Outport
  TH2 : Outport  Port=2
  TH3 : Outport  Port=3
  TH4 : Outport  Port=4
  wires:
  PLT/1 -> Bus Selector6/1
  Bus Selector6/1 -> [PLT]  "<TH_VEL>"
  CMD/1 -> Bus Selector5/1
  Bus Selector5/1 -> [CMD]  "<TH_VEL>"
  [CMD] -> Selector4/1
  Selector1/1 -> Mux/2
  Selector4/1 -> Mux/1
  [PLT] -> Selector1/1
  Mux/1 -> TH1/1
  [CMD] -> Selector3/1
  Selector2/1 -> Mux1/2
  Selector3/1 -> Mux1/1
  [PLT] -> Selector2/1
  Mux1/1 -> TH2/1
  [CMD] -> Selector6/1
  Selector5/1 -> Mux2/2
  Selector6/1 -> Mux2/1
  [PLT] -> Selector5/1
  Mux2/1 -> TH3/1
  [CMD] -> Selector8/1
  Selector7/1 -> Mux3/2
  Selector8/1 -> Mux3/1
  [PLT] -> Selector7/1
  Mux3/1 -> TH4/1

== system bh_4dof_LAGR_manipulator_CONTROL_PID/Create_PLANT_BUS/CALC_BUS ==
  MODEL_BUS : Inport
  Bus Creator : BusCreator  Inputs=14
  Bus Selector : BusSelector  OutputSignals=TH1,TH2,TH3,TH4
  Bus Selector1 : BusSelector  OutputSignals=TH1,TH2,TH3
  Constant1 : Constant  Value=L2y
  Constant17 : Constant  Value=L2y
  Constant18 : Constant  Value=L1y
  Constant19 : Constant  Value=L3y
  Constant2 : Constant  Value=L1y
  Constant3 : Constant  Value=L3y
  THE_A_EFF_and_O_and_G : MATLAB Function  TreatAsAtomicUnit=on
  THE_W_EFF_and_O_and_G : MATLAB Function  TreatAsAtomicUnit=on
  CALC_POS : Outport
  wires:
  Bus Selector/1 -> THE_W_EFF_and_O_and_G/4(theta1)  "<TH1>"
  Bus Selector/2 -> THE_W_EFF_and_O_and_G/5(theta2)  "<TH2>"
  Bus Selector/3 -> THE_W_EFF_and_O_and_G/6(theta3)  "<TH3>"
  Bus Selector/4 -> THE_W_EFF_and_O_and_G/7(theta4)  "<TH4>"
  Bus Creator/1 -> CALC_POS/1
  Constant18/1 -> THE_W_EFF_and_O_and_G/1(L1Y_s)
  Constant17/1 -> THE_W_EFF_and_O_and_G/2(L2Y_s)
  Constant19/1 -> THE_W_EFF_and_O_and_G/3(L3Y_s)
  THE_W_EFF_and_O_and_G/4(WF_pos_O3) -> Bus Creator/4  "WF_pos_O3"
  THE_W_EFF_and_O_and_G/6(WF_pos_G2) -> Bus Creator/6  "WF_pos_G2"
  THE_W_EFF_and_O_and_G/3(WF_pos_O2) -> Bus Creator/3  "WF_pos_O2"
  THE_W_EFF_and_O_and_G/7(WF_pos_G3) -> Bus Creator/7  "WF_pos_G3"
  THE_W_EFF_and_O_and_G/1(WF_pos_eff) -> Bus Creator/1  "WF_pos_EFF"
  THE_W_EFF_and_O_and_G/5(WF_pos_G1) -> Bus Creator/5  "WF_pos_G1"
  THE_W_EFF_and_O_and_G/2(WF_pos_O1) -> Bus Creator/2  "WF_pos_O1"
  MODEL_BUS/1 -> Bus Selector1/1, Bus Selector/1
  Bus Selector1/1 -> THE_A_EFF_and_O_and_G/4(theta1)  "<TH1>"
  Bus Selector1/2 -> THE_A_EFF_and_O_and_G/5(theta2)  "<TH2>"
  Bus Selector1/3 -> THE_A_EFF_and_O_and_G/6(theta3)  "<TH3>"
  Constant2/1 -> THE_A_EFF_and_O_and_G/1(L1Y_s)
  Constant1/1 -> THE_A_EFF_and_O_and_G/2(L2Y_s)
  Constant3/1 -> THE_A_EFF_and_O_and_G/3(L3Y_s)
  THE_A_EFF_and_O_and_G/7(AF_pos_G3) -> Bus Creator/14  "AF_pos_G3"
  THE_A_EFF_and_O_and_G/6(AF_pos_G2) -> Bus Creator/13  "AF_pos_G2"
  THE_A_EFF_and_O_and_G/5(AF_pos_G1) -> Bus Creator/12  "AF_pos_G1"
  THE_A_EFF_and_O_and_G/4(AF_pos_O3) -> Bus Creator/11  "AF_pos_O3"
  THE_A_EFF_and_O_and_G/3(AF_pos_O2) -> Bus Creator/10  "AF_pos_O2"
  THE_A_EFF_and_O_and_G/2(AF_pos_O1) -> Bus Creator/9  "AF_pos_O1"
  THE_A_EFF_and_O_and_G/1(AF_pos_eff) -> Bus Creator/8  "AF_pos_EFF"

== system bh_4dof_LAGR_manipulator_CONTROL_PID/Create_PLANT_BUS/MEAS ==
  MODEL_BUS : Inport
  Bus Creator : BusCreator  Inputs=3
  Bus Selector : BusSelector  OutputSignals=TH1,TH2,TH3,TH4
  Bus Selector1 : BusSelector  OutputSignals=TH1_D,TH2_D,TH3_D,TH4_D
  Bus Selector2 : BusSelector  OutputSignals=TH1_DD,TH2_DD,TH3_DD,TH4_DD
  Mux : Mux
  Mux1 : Mux
  Mux2 : Mux
  Reshape : Reshape  OutputDimensionality=Column vector (2-D)
  Reshape1 : Reshape  OutputDimensionality=Column vector (2-D)
  Reshape2 : Reshape  OutputDimensionality=Column vector (2-D)
  MEAS : Outport
  wires:
  MODEL_BUS/1 -> Bus Selector/1, Bus Selector2/1, Bus Selector1/1
  Bus Selector/1 -> Mux/1  "<TH1>"
  Bus Selector/2 -> Mux/2  "<TH2>"
  Bus Selector/3 -> Mux/3  "<TH3>"
  Bus Selector/4 -> Mux/4  "<TH4>"
  Bus Selector1/1 -> Mux1/1  "<TH1_D>"
  Bus Selector1/2 -> Mux1/2  "<TH2_D>"
  Bus Selector1/3 -> Mux1/3  "<TH3_D>"
  Bus Selector1/4 -> Mux1/4  "<TH4_D>"
  Bus Selector2/1 -> Mux2/1  "<TH1_DD>"
  Bus Selector2/2 -> Mux2/2  "<TH2_DD>"
  Bus Selector2/3 -> Mux2/3  "<TH3_DD>"
  Bus Selector2/4 -> Mux2/4  "<TH4_DD>"
  Mux/1 -> Reshape/1  "TH_POS"
  Mux1/1 -> Reshape1/1  "TH_VEL"
  Mux2/1 -> Reshape2/1  "TH_ACC"
  Reshape/1 -> Bus Creator/1  "TH_POS"
  Reshape1/1 -> Bus Creator/2  "TH_VEL"
  Reshape2/1 -> Bus Creator/3  "TH_ACC"
  Bus Creator/1 -> MEAS/1

== system bh_4dof_LAGR_manipulator_CONTROL_PID/Create_PLANT_BUS/Subsystem ==
  MODEL : Inport
  MEAS : Inport  Port=2
  CALC_POS : Inport  Port=3
  CALC_GRAV_TQ : Inport  Port=4
  Bus Creator : BusCreator  Inputs=4
  PLANT_B : Outport
  wires:
  MODEL/1 -> Bus Creator/1  "MODEL_BUS"
  MEAS/1 -> Bus Creator/2  "MEAS_BUS"
  CALC_POS/1 -> Bus Creator/3  "CALC_POS_BUS"
  Bus Creator/1 -> PLANT_B/1
  CALC_GRAV_TQ/1 -> Bus Creator/4  "CALC_GRAV_TQ_BUS"

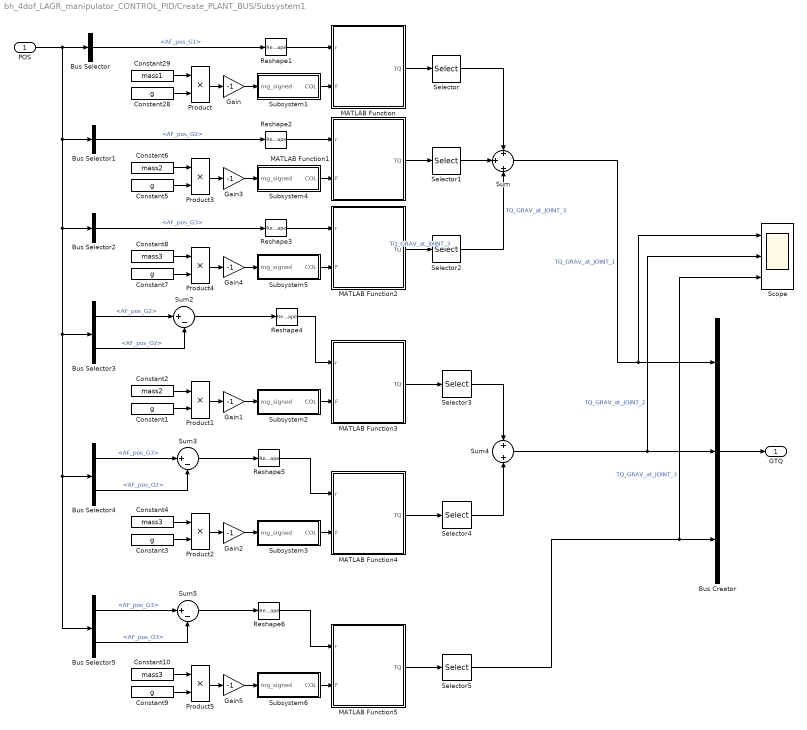
== system bh_4dof_LAGR_manipulator_CONTROL_PID/Create_PLANT_BUS/Subsystem1 ==
  POS : Inport
  Bus Creator : BusCreator  Inputs=3
  Bus Selector : BusSelector  OutputSignals=AF_pos_G1
  Bus Selector1 : BusSelector  OutputSignals=AF_pos_G2
  Bus Selector2 : BusSelector  OutputSignals=AF_pos_G3
  Bus Selector3 : BusSelector  OutputSignals=AF_pos_G2,AF_pos_O2
  Bus Selector4 : BusSelector  OutputSignals=AF_pos_G3,AF_pos_O2
  Bus Selector5 : BusSelector  OutputSignals=AF_pos_G3,AF_pos_O3
  Constant{1,3,5,7,9,28} (6 alike) : Constant  Value=g
  Constant10 : Constant  Value=mass3
  Constant2 : Constant  Value=mass2
  Constant29 : Constant  Value=mass1
  Constant4 : Constant  Value=mass3
  Constant6 : Constant  Value=mass2
  Constant8 : Constant  Value=mass3
  Gain{,1..5} (6 alike) : Gain  Gain=-1
  MATLAB Function : MATLAB Function  TreatAsAtomicUnit=on
  MATLAB Function1 : MATLAB Function  TreatAsAtomicUnit=on
  MATLAB Function2 : MATLAB Function  TreatAsAtomicUnit=on
  MATLAB Function3 : MATLAB Function  TreatAsAtomicUnit=on
  MATLAB Function4 : MATLAB Function  TreatAsAtomicUnit=on
  MATLAB Function5 : MATLAB Function  TreatAsAtomicUnit=on
  Product{,1..5} (6 alike) : Product
  Reshape{1..6} (6 alike) : Reshape  OutputDimensionality=Column vector (2-D)
  Scope : Scope  NumInputPorts=3
  Selector{,1..5} (6 alike) : Selector  InputPortWidth=3  IndexOptions=Index vector (dialog)  Indices=1  OutputSizes=1
  Subsystem1 : Subsystem
  Subsystem2 : Subsystem
  Subsystem3 : Subsystem
  Subsystem4 : Subsystem
  Subsystem5 : Subsystem
  Subsystem6 : Subsystem
  Sum : Sum  Inputs=+|+|+
  Sum2 : Sum  Inputs=|+-
  Sum3 : Sum  Inputs=|+-
  Sum4 : Sum  Inputs=+|+
  Sum5 : Sum  Inputs=|+-
  GTQ : Outport
  wires:
  Bus Selector/1 -> Reshape1/1  "<AF_pos_G1>"
  Constant29/1 -> Product/1
  Constant28/1 -> Product/2
  Product/1 -> Gain/1
  Gain/1 -> Subsystem1/1(mg_signed)
  Subsystem1/1(COL) -> MATLAB Function/2(F)
  Reshape1/1 -> MATLAB Function/1(r)
  Bus Selector1/1 -> Reshape2/1  "<AF_pos_G2>"
  Constant6/1 -> Product3/1
  Constant5/1 -> Product3/2
  Product3/1 -> Gain3/1
  Gain3/1 -> Subsystem4/1(mg_signed)
  Subsystem4/1(COL) -> MATLAB Function1/2(F)
  Reshape2/1 -> MATLAB Function1/1(r)
  Bus Selector2/1 -> Reshape3/1  "<AF_pos_G3>"
  Constant8/1 -> Product4/1
  Constant7/1 -> Product4/2
  Product4/1 -> Gain4/1
  Gain4/1 -> Subsystem5/1(mg_signed)
  Subsystem5/1(COL) -> MATLAB Function2/2(F)
  Reshape3/1 -> MATLAB Function2/1(r)
  MATLAB Function/1(TQ) -> Selector/1
  MATLAB Function2/1(TQ) -> Selector2/1  "TQ_GRAV_at_JOINT_3"
  MATLAB Function1/1(TQ) -> Selector1/1
  Bus Creator/1 -> GTQ/1
  Selector/1 -> Sum/1
  Selector1/1 -> Sum/2
  Selector2/1 -> Sum/3  "TQ_GRAV_at_JOINT_3"
  Bus Selector3/1 -> Sum2/1  "<AF_pos_G2>"
  Constant2/1 -> Product1/1
  Constant1/1 -> Product1/2
  Product1/1 -> Gain1/1
  Gain1/1 -> Subsystem2/1(mg_signed)
  Subsystem2/1(COL) -> MATLAB Function3/2(F)
  Reshape4/1 -> MATLAB Function3/1(r)
  Bus Selector4/1 -> Sum3/1  "<AF_pos_G3>"
  Constant4/1 -> Product2/1
  Constant3/1 -> Product2/2
  Product2/1 -> Gain2/1
  Gain2/1 -> Subsystem3/1(mg_signed)
  Subsystem3/1(COL) -> MATLAB Function4/2(F)
  Reshape5/1 -> MATLAB Function4/1(r)
  Sum2/1 -> Reshape4/1
  Bus Selector3/2 -> Sum2/2  "<AF_pos_O2>"
  Bus Selector4/2 -> Sum3/2  "<AF_pos_O2>"
  Sum3/1 -> Reshape5/1
  MATLAB Function3/1(TQ) -> Selector3/1
  MATLAB Function4/1(TQ) -> Selector4/1
  Selector3/1 -> Sum4/1
  Selector4/1 -> Sum4/2
  POS/1 -> Bus Selector5/1, Bus Selector4/1, Bus Selector3/1, Bus Selector2/1, Bus Selector1/1, Bus Selector/1
  Bus Selector5/1 -> Sum5/1  "<AF_pos_G3>"
  Constant10/1 -> Product5/1
  Constant9/1 -> Product5/2
  Product5/1 -> Gain5/1
  Gain5/1 -> Subsystem6/1(mg_signed)
  Subsystem6/1(COL) -> MATLAB Function5/2(F)
  Reshape6/1 -> MATLAB Function5/1(r)
  Bus Selector5/2 -> Sum5/2  "<AF_pos_O3>"
  Sum5/1 -> Reshape6/1
  MATLAB Function5/1(TQ) -> Selector5/1
  Sum4/1 -> Scope/2, Bus Creator/2  "TQ_GRAV_at_JOINT_2"
  Sum/1 -> Scope/1, Bus Creator/1  "TQ_GRAV_at_JOINT_1"
  Selector5/1 -> Scope/3, Bus Creator/3  "TQ_GRAV_at_JOINT_3"

== system bh_4dof_LAGR_manipulator_CONTROL_PID/TRAJECTORY/End_Eff_Traj ==
  Bus Creator : BusCreator  Inputs=8
  Demux : Demux  Outputs=3
  Demux1 : Demux  Outputs=3
  From Spreadsheet : FromSpreadsheet  FileName=bh_hello_complete.xlsx  SheetName=COMP_SPLINE _4dof  SampleTime=0.1  ExtrapolationBeforeFirstDataPoint=Hold first value  ExtrapolationAfterLastDataPoint=Hold last value
  Mux : Mux  Inputs=3
  Mux1 : Mux  Inputs=3
  Reshape : Reshape  OutputDimensionality=Column vector (2-D)
  Reshape1 : Reshape  OutputDimensionality=Column vector (2-D)
  EFF_TRAJ : Outport
  wires:
  From Spreadsheet/2 -> Mux/2  "YE"
  From Spreadsheet/3 -> Mux/3  "ZE"
  From Spreadsheet/1 -> Mux/1  "XE"
  From Spreadsheet/4 -> Mux1/1  "DXEDT"
  Bus Creator/1 -> EFF_TRAJ/1
  From Spreadsheet/6 -> Mux1/3  "DZEDT"
  From Spreadsheet/5 -> Mux1/2  "DYEDT"
  Demux/1 -> Bus Creator/6  "DXEDT"
  Demux/2 -> Bus Creator/7  "DYEDT"
  Demux/3 -> Bus Creator/8  "DZEDT"
  Demux1/1 -> Bus Creator/1  "XE"
  Demux1/2 -> Bus Creator/2  "YE"
  Demux1/3 -> Bus Creator/3  "ZE"
  Mux/1 -> Reshape/1  "XYZ"
  Mux1/1 -> Reshape1/1
  Reshape/1 -> Bus Creator/4, Demux1/1  "XYZ_POS"
  Reshape1/1 -> Demux/1, Bus Creator/5  "XYZ_VEL"

== system bh_4dof_LAGR_manipulator_CONTROL_PID/TRAJECTORY/Subsystem ==
  In1 : Inport
  In2 : Inport  Port=2
  Mux2 : Mux  Inputs=2
  Reshape : Reshape  OutputDimensionality=Column vector (2-D)
  Reshape1 : Reshape  OutputDimensionality=Column vector (2-D)
  Selector : Selector  InputPortWidth=8  IndexOptions=Index vector (dialog)  Indices=[1 5]  OutputSizes=1
  Selector1 : Selector  InputPortWidth=8  IndexOptions=Index vector (dialog)  Indices=[2 6]  OutputSizes=1
  Selector2 : Selector  InputPortWidth=8  IndexOptions=Index vector (dialog)  Indices=[3 7]  OutputSizes=1
  Selector3 : Selector  InputPortWidth=8  IndexOptions=Index vector (dialog)  Indices=[4 8]  OutputSizes=1
  Out1 : Outport
  Out2 : Outport  Port=2
  Out3 : Outport  Port=3
  Out4 : Outport  Port=4
  wires:
  In1/1 -> Reshape/1
  In2/1 -> Reshape1/1
  Reshape/1 -> Mux2/1
  Reshape1/1 -> Mux2/2
  Selector2/1 -> Out3/1
  Selector1/1 -> Out2/1
  Selector/1 -> Out1/1
  Mux2/1 -> Selector1/1, Selector/1, Selector2/1, Selector3/1
  Selector3/1 -> Out4/1

== system bh_4dof_LAGR_manipulator_CONTROL_PID/TRAJECTORY/XY_compare ==
  XY_GOAL : Inport
  XY : Inport  Port=2
  Bus Selector1 : BusSelector  OutputSignals=XE,YE,ZE
  Demux : Demux  Outputs=3
  Mux : Mux  Inputs=2
  Mux1 : Mux  Inputs=2
  Mux2 : Mux  Inputs=2
  X : Outport
  Y : Outport  Port=2
  Z : Outport  Port=3
  wires:
  XY_GOAL/1 -> Bus Selector1/1
  XY/1 -> Demux/1
  Bus Selector1/1 -> Mux/1  "<XE>"
  Demux/1 -> Mux/2
  Bus Selector1/2 -> Mux1/1  "<YE>"
  Demux/2 -> Mux1/2
  Mux/1 -> X/1
  Mux1/1 -> Y/1
  Mux2/1 -> Z/1
  Bus Selector1/3 -> Mux2/1  "<ZE>"
  Demux/3 -> Mux2/2

== system bh_4dof_LAGR_manipulator_CONTROL_PID/TRAJECTORY/get_XYDOT ==
  In1 : Inport
  Bus Selector2 : BusSelector  OutputSignals=DXEDT,DYEDT,DZEDT
  Mux2 : Mux  Inputs=3
  Reshape : Reshape  OutputDimensionality=Column vector (2-D)
  Out1 : Outport
  wires:
  Bus Selector2/1 -> Mux2/1  "<DXEDT>"
  Bus Selector2/2 -> Mux2/2  "<DYEDT>"
  In1/1 -> Bus Selector2/1
  Mux2/1 -> Reshape/1
  Reshape/1 -> Out1/1  "XY_DOT"
  Bus Selector2/3 -> Mux2/3  "<DZEDT>"

== system bh_4dof_LAGR_manipulator_CONTROL_PID/VIEW/XYZ_EFF_COMPARE1 ==
  CMD_BUS : Inport
  PLANT_BUS : Inport  Port=2
  Bus Selector1 : BusSelector  OutputSignals=CALC_POS_BUS.WF_pos_EFF
  Bus Selector4 : BusSelector  OutputSignals=XYZ_BUS.XYZ_POS
  Mux : Mux  Inputs=2
  Reshape1 : Reshape  OutputDimensionality=Column vector (2-D)
  Reshape2 : Reshape  OutputDimensionality=Column vector (2-D)
  Selector : Selector  InputPortWidth=6  IndexOptions=Index vector (dialog)  Indices=[1 4]  OutputSizes=1
  Selector1 : Selector  InputPortWidth=6  IndexOptions=Index vector (dialog)  Indices=[2 5]  OutputSizes=1
  Selector2 : Selector  InputPortWidth=6  IndexOptions=Index vector (dialog)  Indices=[3 6]  OutputSizes=1
  X : Outport
  Y : Outport  Port=2
  Z : Outport  Port=3
  wires:
  CMD_BUS/1 -> Bus Selector4/1
  PLANT_BUS/1 -> Bus Selector1/1
  Bus Selector4/1 -> Reshape1/1  "<XYZ_POS>"
  Bus Selector1/1 -> Reshape2/1  "<WF_pos_EFF>"
  Reshape1/1 -> Mux/1
  Reshape2/1 -> Mux/2
  Mux/1 -> Selector2/1, Selector1/1, Selector/1
  Selector2/1 -> Z/1
  Selector1/1 -> Y/1
  Selector/1 -> X/1
